simulink model "test_ref"  (R2019b)
settings: Solver=VariableStepAuto  StartTime=0.0  StopTime=simTime  RelTol=1e-3
values from neighbouring files (symbols this model uses):
  x0 = [L2;0;0;0;0;0]    [initHaloSRMPC.m]
settings Model: Creator=mohd-  LastModifiedBy=mohd-

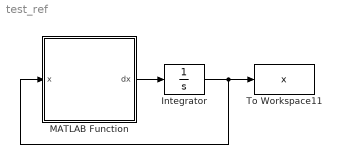
== system test_ref ==
  Integrator : Integrator  InitialCondition=x0
  MATLAB Function : MATLAB Function  TreatAsAtomicUnit=on
  To Workspace11 : ToWorkspace  VariableName=x  SampleTime=10^-3
  wires:
  MATLAB Function/1(dx) -> Integrator/1
  Integrator/1 -> To Workspace11/1, MATLAB Function/1(x)

== matlab function test_ref/MATLAB Function ==
  data: x input; dx output; A parameter
function dx = fcn(x,A)

dx = A*x;
